simulink model "arduino_lab_mhe_R2015a"  (R2015a)
settings: Solver=ode45  StartTime=0.0  StopTime=500  RelTol=1e-3
StartFcn:
  | clear all
libraries: simulink x1, realtime_pacer_lib x1
settings Model: Creator=johnh  LastModifiedBy=johnh
settings DataIOCC: LimitDataPoints=off  SaveFormat=Dataset
settings HardwareCC: ProdBitPerPointer=64  ProdLargestAtomicFloat=Float  ProdIntDivRoundTo=Zero  ProdEndianess=LittleEndian  ProdHWDeviceType=Specified
settings ModelReferenceCC: PropagateSignalLabelsOutOfModel=on

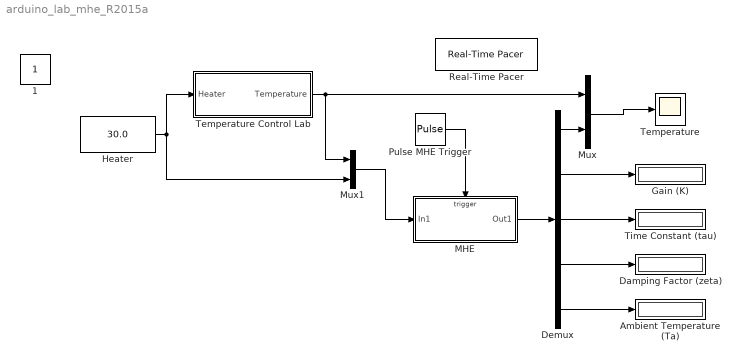
== system arduino_lab_mhe_R2015a ==
  Ambient Temperature (Ta) : Display
      settings: Decimation=2
  Damping Factor (zeta) : Display
      settings: Decimation=2
  Demux : Demux  Outputs=5
  Gain (K) : Display
      settings: Decimation=2
  Heater : simulink/Math Operations/Slider Gain  gain=30.0  low=0  high=100
  MHE : Subsystem  TreatAsAtomicUnit=on
  Mux : Mux  Inputs=2
  Mux1 : Mux  Inputs=2
  Pulse MHE Trigger : DiscretePulseGenerator  PulseType=Time based  PulseWidth=5
  Real-Time Pacer : realtime_pacer_lib/Real-Time Pacer  simTimePerRealTime=1
  Temperature : Scope
      settings: TimeRange=auto  MaxDataPoints=5000  SaveToWorkspace=off  YMin=18.64675  YMax=62.17925  SampleTime=-1
  Temperature Control Lab : Subsystem
  Time Constant (tau) : Display
      settings: Decimation=2
  1 : Constant  IOType=siggen
  wires:
  Temperature Control Lab/1(Temperature) -> Mux1/1, Mux/1
  Heater/1 -> Temperature Control Lab/1(Heater), Mux1/2
  Pulse MHE Trigger/1 -> MHE/Trigger
  Mux1/1 -> MHE/1(In1)
  MHE/1(Out1) -> Demux/1
  Mux/1 -> Temperature/1
  Demux/1 -> Mux/2
  Demux/2 -> Gain (K)/1
  Demux/3 -> Time Constant (tau)/1
  Demux/4 -> Damping Factor (zeta)/1
  Demux/5 -> Ambient Temperature (Ta)/1

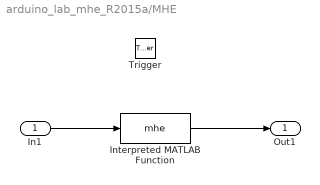
== system arduino_lab_mhe_R2015a/MHE ==
  In1 : Inport  LatchByDelayingOutsideSignal=on
  Trigger : TriggerPort
  Interpreted MATLAB Function : MATLABFcn  MATLABFcn=mhe  OutputDimensions=5
  Out1 : Outport  InitialOutput=[23 0.5 50 1.5 23]
  wires:
  In1/1 -> Interpreted MATLAB Function/1
  Interpreted MATLAB Function/1 -> Out1/1

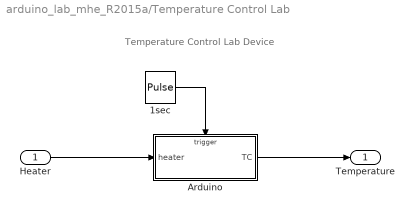
== system arduino_lab_mhe_R2015a/Temperature Control Lab ==
  note: Temperature Control Lab Device
  Heater : Inport
  1sec : DiscretePulseGenerator  PulseType=Time based  Period=1  PulseWidth=50
  Arduino : Subsystem  TreatAsAtomicUnit=on
  Temperature : Outport
  wires:
  1sec/1 -> Arduino/Trigger
  Arduino/1(TC) -> Temperature/1
  Heater/1 -> Arduino/1(heater)

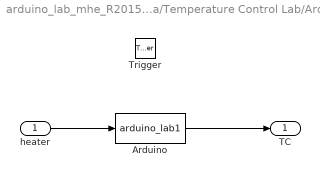
== system arduino_lab_mhe_R2015a/Temperature Control Lab/Arduino ==
  heater : Inport  LatchByDelayingOutsideSignal=on
  Trigger : TriggerPort
  Arduino : MATLABFcn  MATLABFcn=arduino_lab1
  TC : Outport  InitialOutput=23
  wires:
  heater/1 -> Arduino/1
  Arduino/1 -> TC/1
